simulink model "dupla_estrela_filtro_harmonico_Daniel_13mvar"  (R2023a)
settings: Solver=VariableStepAuto  StartTime=0.0  StopTime=10  FixedStep=1e-6
InitFcn:
  | r = 0.001
  | 
  | f1 = 60
  | w1 = 2 * pi * f1
  | power_bank = 13*1e6
  | voltage_bank = 34.5*1e3
  | current_bank = power_bank / (sqrt(3)*voltage_bank)
  | reactance_bank = voltage_bank^2 / power_bank
  | capacitance_bank = 1 / (w1*reactance_bank)
  | 
  | capacitance_branch = capacitance_bank / 2
  | 
  | N = 9
  | Su = 5
  | S = 2
  | 
  | C = capacitance_branch * S
  | c = C * Su / N
  | 
  | R = r * Su / N
libraries: spsSeriesRLCBranchLib x52, spsVoltageMeasurementLib x4, spsCurrentMeasurementLib x2, spsGroundLib x1, spsRMSLib x1, spsThreePhaseSourceLib x1, spspowerguiLib x1
settings Model: Creator=angel  LastModifiedBy=angel

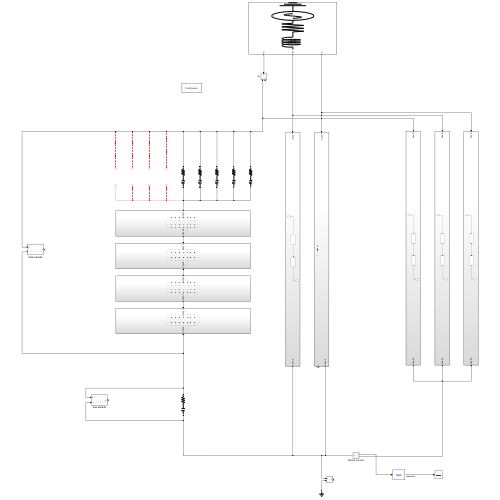
[thumbnail: Simulink's stored preview of the top-level diagram]
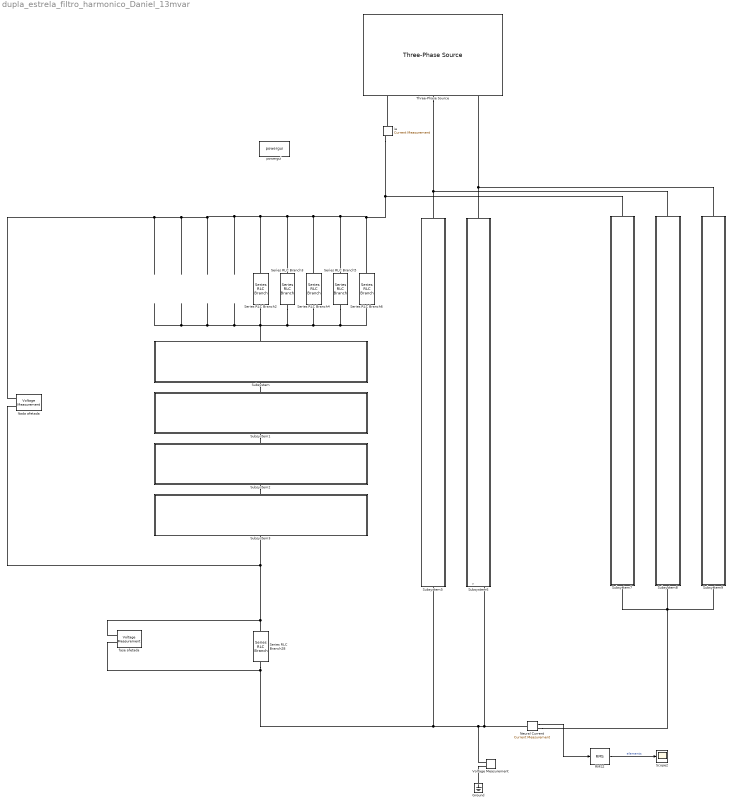
== system dupla_estrela_filtro_harmonico_Daniel_13mvar ==
  Ground : spsGroundLib/Ground  LConnTagsString=a
  Neural Current : spsCurrentMeasurementLib/Current Measurement  PhasorSimulation=off  OutputType=Complex  PSBequivalent=0
  RMS2 : spsRMSLib/RMS  TrueRMS=on  Freq=60  RMSInit=0  Ts=0
  Scope2 : Scope
  Series RLC Branch{2..6} (5 alike) : spsSeriesRLCBranchLib/Series RLC Branch  LConnTagsString=__new0  RConnTagsString=__new0  BranchType=RC  Resistance=r  Inductance=0  SetiL0=off  InitialCurrent=0  Capacitance=c  Setx0=off  InitialVoltage=0  Measurements=None
  Series RLC Branch28 : spsSeriesRLCBranchLib/Series RLC Branch  LConnTagsString=__new0  RConnTagsString=__new0  BranchType=RC  Resistance=R  Inductance=0  SetiL0=off  InitialCurrent=0  Capacitance=C  Setx0=off  InitialVoltage=0  Measurements=None
  Subsystem : Subsystem
  Subsystem1 : Subsystem
  Subsystem2 : Subsystem
  Subsystem3 : Subsystem
  Subsystem5 : Subsystem
  Subsystem6 : Subsystem
  Subsystem7 : Subsystem
  Subsystem8 : Subsystem
  Subsystem9 : Subsystem
  Three-Phase Source : spsThreePhaseSourceLib/Three-Phase Source  InternalConnection=Yg  VoltagePhases=off  Voltage=voltage_bank  PhaseAngle=0  Voltage_phases=[25e3 25e3 25e3]/sqrt(3)  PhaseAngles_phases=[0 -120 +120]  Frequency=60  NonIdealSource=on  SpecifyImpedance=off  Resistance=0.8929  Inductance=16.58e-6  ShortCircuitLevel=100e6  BaseVoltage=voltage_bank  XRratio=7  BusType=swing  Pref=10e3  Qref=0  Prefabc=[10e3, 10e3, 10e3]  Qrefabc=[0, 0, 0]  Qmin=-inf  Qmax=inf
  Voltage Measurement : spsVoltageMeasurementLib/Voltage Measurement  PhasorSimulation=off  OutputType=Complex  PSBequivalent=0
  fase afetada : spsVoltageMeasurementLib/Voltage Measurement  PhasorSimulation=off  OutputType=Complex  PSBequivalent=0
  ia : spsCurrentMeasurementLib/Current Measurement  PhasorSimulation=off  OutputType=Complex  PSBequivalent=0
  ltada afetada : spsVoltageMeasurementLib/Voltage Measurement  PhasorSimulation=off  OutputType=Complex  PSBequivalent=0
  powergui : spspowerguiLib/powergui  Priority=1  SimulationMode=Continuous  SampleTime=50e-6  frequency=60  Iterations=50  frequencyindice=60  Pbase=100e6  ErrMax=1e-4  UnitsV=kV  UnitsW=MW  buscounter=0  FunctionMessages=off  echomessages=off  EnableUseOfTLC=off  CurrentSourceSwitches=off  DisableSnubberDevices=off  DisableRonSwitches=off  DisableVfSwitches=off  DisplayEquations=off  AutomaticDiscreteSolvers=off  SolverType=Tustin/Backward Euler (TBE)  Interpol=off  ExternalGateDelay=off  methode=off  Ts=100  x0status=blocks  SPID=on  SwTol=0  HookPort=off  NonlinearTolerance=1e-4  nMaxIteration=100  ContinueOnMaxIteration=off  RestoreLinks=warning  ResistiveCurrentMeasurement=off  Frange=[0:2:500]  Ylog=off  Xlog=on  ShowGrid=off  save=off  variable=ZData  structure=0  ZoomFFT=off  StartTime=0.0  cycles=1  DisplayStyle=1  fundamental=60  FreqAxis=off  MaxFrequency=1000  frequencyindicesteady=1  RmsSteady=1  display=off
  wires:
  Neural Current/1 -> RMS2/1
  RMS2/1 -> Scope2/1  "elements"
  connections:
  Series RLC Branch6/RConn1 -- Series RLC Branch5/RConn1 -- Series RLC Branch4/RConn1 -- Series RLC Branch3/RConn1 -- Subsystem/LConn1 -- Series RLC Branch2/RConn1
  ltada afetada/LConn1 -- Series RLC Branch2/LConn1 -- Series RLC Branch3/LConn1 -- Series RLC Branch4/LConn1 -- Series RLC Branch5/LConn1 -- Subsystem7/LConn1 -- ia/RConn1 -- Series RLC Branch6/LConn1
  Three-Phase Source/RConn2 -- Subsystem8/LConn1 -- Subsystem5/LConn1
  fase afetada/LConn2 -- Series RLC Branch28/RConn1 -- Subsystem5/RConn1 -- Subsystem6/RConn1 -- Neural Current/LConn1 -- Voltage Measurement/LConn1
  Subsystem/RConn1 -- Subsystem1/LConn1
  Subsystem1/RConn1 -- Subsystem2/LConn1
  Subsystem2/RConn1 -- Subsystem3/LConn1
  Series RLC Branch28/LConn1 -- ltada afetada/LConn2 -- Subsystem3/RConn1 -- fase afetada/LConn1
  Three-Phase Source/RConn3 -- Subsystem6/LConn1 -- Subsystem9/LConn1
  Neural Current/RConn1 -- Subsystem9/RConn1 -- Subsystem8/RConn1 -- Subsystem7/RConn1
  ia/LConn1 -- Three-Phase Source/RConn1
  Ground/LConn1 -- Voltage Measurement/LConn2

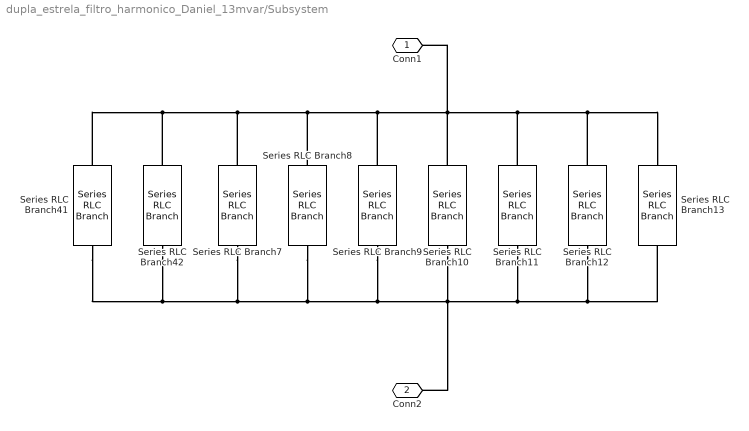
== system dupla_estrela_filtro_harmonico_Daniel_13mvar/Subsystem ==
  Series RLC Branch{7..13,41..42} (9 alike) : spsSeriesRLCBranchLib/Series RLC Branch  LConnTagsString=__new0  RConnTagsString=__new0  BranchType=RC  Resistance=r  Inductance=0  SetiL0=off  InitialCurrent=0  Capacitance=c  Setx0=off  InitialVoltage=0  Measurements=None
  Conn1 : PMIOPort  Side=Left
  Conn2 : PMIOPort  Port=2  Side=Right
  connections:
  Series RLC Branch42/LConn1 -- Series RLC Branch8/LConn1 -- Series RLC Branch9/LConn1 -- Conn1/RConn1 -- Series RLC Branch11/LConn1 -- Series RLC Branch12/LConn1 -- Series RLC Branch13/LConn1 -- Series RLC Branch10/LConn1 -- Series RLC Branch7/LConn1 -- Series RLC Branch41/LConn1
  Series RLC Branch42/RConn1 -- Series RLC Branch7/RConn1 -- Conn2/RConn1 -- Series RLC Branch13/RConn1 -- Series RLC Branch12/RConn1 -- Series RLC Branch11/RConn1 -- Series RLC Branch10/RConn1 -- Series RLC Branch9/RConn1 -- Series RLC Branch8/RConn1 -- Series RLC Branch41/RConn1

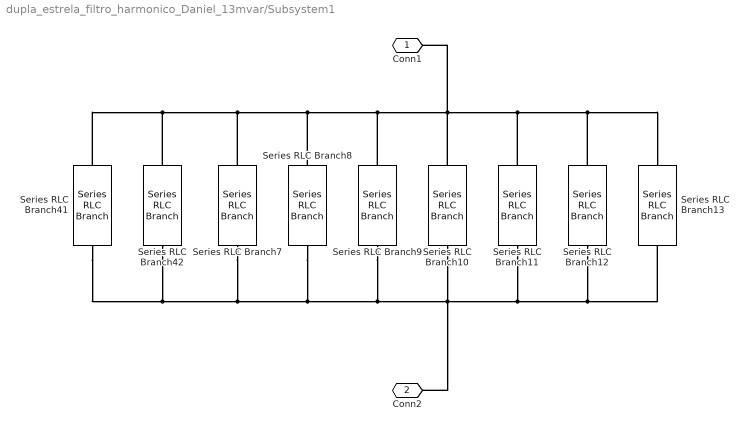
== system dupla_estrela_filtro_harmonico_Daniel_13mvar/Subsystem1 ==
  Series RLC Branch{7..13,41..42} (9 alike) : spsSeriesRLCBranchLib/Series RLC Branch  LConnTagsString=__new0  RConnTagsString=__new0  BranchType=RC  Resistance=r  Inductance=0  SetiL0=off  InitialCurrent=0  Capacitance=c  Setx0=off  InitialVoltage=0  Measurements=None
  Conn1 : PMIOPort  Side=Left
  Conn2 : PMIOPort  Port=2  Side=Right
  connections:
  Conn2/RConn1 -- Series RLC Branch10/RConn1 -- Series RLC Branch9/RConn1 -- Series RLC Branch8/RConn1 -- Series RLC Branch42/RConn1 -- Series RLC Branch41/RConn1 -- Series RLC Branch7/RConn1 -- Series RLC Branch11/RConn1 -- Series RLC Branch12/RConn1 -- Series RLC Branch13/RConn1
  Conn1/RConn1 -- Series RLC Branch10/LConn1 -- Series RLC Branch13/LConn1 -- Series RLC Branch12/LConn1 -- Series RLC Branch11/LConn1 -- Series RLC Branch9/LConn1 -- Series RLC Branch8/LConn1 -- Series RLC Branch7/LConn1 -- Series RLC Branch41/LConn1 -- Series RLC Branch42/LConn1

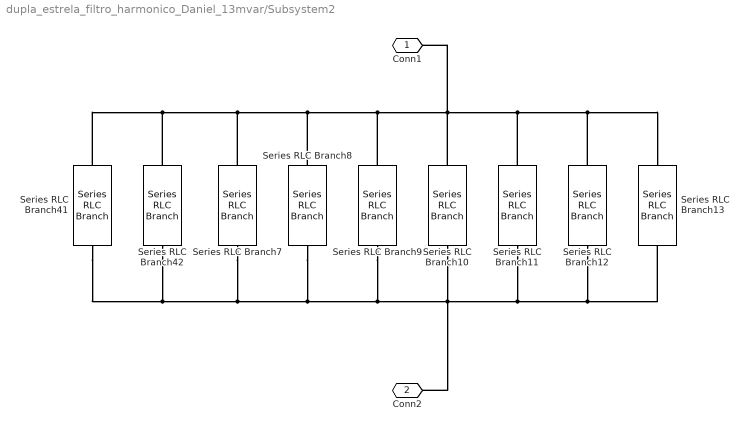
== system dupla_estrela_filtro_harmonico_Daniel_13mvar/Subsystem2 ==
  Series RLC Branch{7..13,41..42} (9 alike) : spsSeriesRLCBranchLib/Series RLC Branch  LConnTagsString=__new0  RConnTagsString=__new0  BranchType=RC  Resistance=r  Inductance=0  SetiL0=off  InitialCurrent=0  Capacitance=c  Setx0=off  InitialVoltage=0  Measurements=None
  Conn1 : PMIOPort  Side=Left
  Conn2 : PMIOPort  Port=2  Side=Right
  connections:
  Series RLC Branch42/LConn1 -- Series RLC Branch41/LConn1 -- Series RLC Branch7/LConn1 -- Series RLC Branch8/LConn1 -- Series RLC Branch9/LConn1 -- Series RLC Branch11/LConn1 -- Series RLC Branch12/LConn1 -- Series RLC Branch13/LConn1 -- Series RLC Branch10/LConn1 -- Conn1/RConn1
  Series RLC Branch13/RConn1 -- Series RLC Branch12/RConn1 -- Series RLC Branch11/RConn1 -- Series RLC Branch7/RConn1 -- Series RLC Branch41/RConn1 -- Series RLC Branch42/RConn1 -- Series RLC Branch8/RConn1 -- Series RLC Branch9/RConn1 -- Series RLC Branch10/RConn1 -- Conn2/RConn1

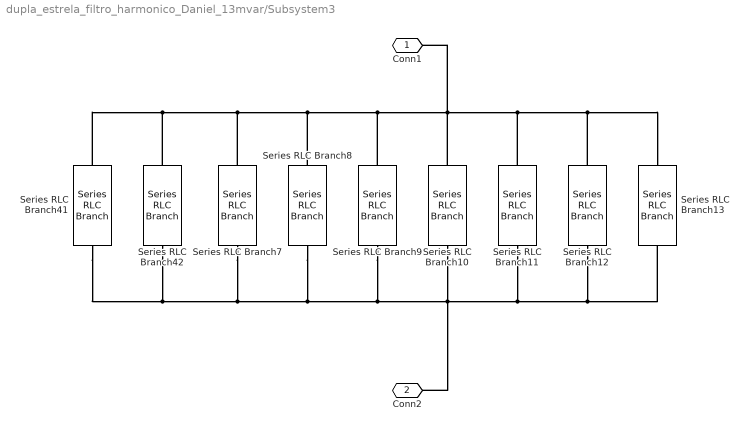
== system dupla_estrela_filtro_harmonico_Daniel_13mvar/Subsystem3 ==
  Series RLC Branch{7..13,41..42} (9 alike) : spsSeriesRLCBranchLib/Series RLC Branch  LConnTagsString=__new0  RConnTagsString=__new0  BranchType=RC  Resistance=r  Inductance=0  SetiL0=off  InitialCurrent=0  Capacitance=c  Setx0=off  InitialVoltage=0  Measurements=None
  Conn1 : PMIOPort  Side=Left
  Conn2 : PMIOPort  Port=2  Side=Right
  connections:
  Conn2/RConn1 -- Series RLC Branch10/RConn1 -- Series RLC Branch9/RConn1 -- Series RLC Branch8/RConn1 -- Series RLC Branch42/RConn1 -- Series RLC Branch41/RConn1 -- Series RLC Branch7/RConn1 -- Series RLC Branch11/RConn1 -- Series RLC Branch12/RConn1 -- Series RLC Branch13/RConn1
  Conn1/RConn1 -- Series RLC Branch10/LConn1 -- Series RLC Branch13/LConn1 -- Series RLC Branch12/LConn1 -- Series RLC Branch11/LConn1 -- Series RLC Branch9/LConn1 -- Series RLC Branch8/LConn1 -- Series RLC Branch7/LConn1 -- Series RLC Branch41/LConn1 -- Series RLC Branch42/LConn1

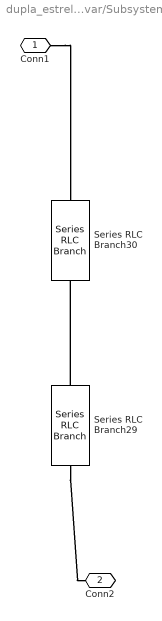
== system dupla_estrela_filtro_harmonico_Daniel_13mvar/Subsystem5 ==
  Series RLC Branch29 : spsSeriesRLCBranchLib/Series RLC Branch  LConnTagsString=__new0  RConnTagsString=__new0  BranchType=RC  Resistance=R  Inductance=0  SetiL0=off  InitialCurrent=0  Capacitance=C  Setx0=off  InitialVoltage=0  Measurements=None
  Series RLC Branch30 : spsSeriesRLCBranchLib/Series RLC Branch  LConnTagsString=__new0  RConnTagsString=__new0  BranchType=RC  Resistance=R  Inductance=0  SetiL0=off  InitialCurrent=0  Capacitance=C  Setx0=off  InitialVoltage=0  Measurements=None
  Conn1 : PMIOPort  Side=Left
  Conn2 : PMIOPort  Port=2  Side=Right
  connections:
  Series RLC Branch29/LConn1 -- Series RLC Branch30/RConn1
  Series RLC Branch29/RConn1 -- Conn2/RConn1
  Conn1/RConn1 -- Series RLC Branch30/LConn1

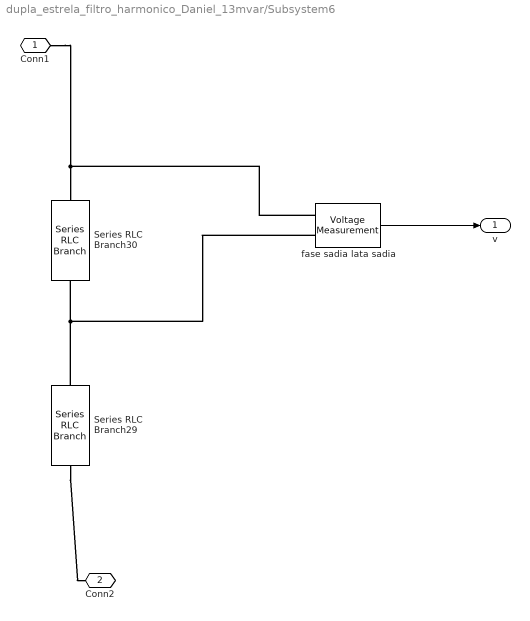
== system dupla_estrela_filtro_harmonico_Daniel_13mvar/Subsystem6 ==
  Series RLC Branch29 : spsSeriesRLCBranchLib/Series RLC Branch  LConnTagsString=__new0  RConnTagsString=__new0  BranchType=RC  Resistance=R  Inductance=0  SetiL0=off  InitialCurrent=0  Capacitance=C  Setx0=off  InitialVoltage=0  Measurements=None
  Series RLC Branch30 : spsSeriesRLCBranchLib/Series RLC Branch  LConnTagsString=__new0  RConnTagsString=__new0  BranchType=RC  Resistance=R  Inductance=0  SetiL0=off  InitialCurrent=0  Capacitance=C  Setx0=off  InitialVoltage=0  Measurements=None
  fase sadia lata sadia : spsVoltageMeasurementLib/Voltage Measurement  PhasorSimulation=off  OutputType=Complex  PSBequivalent=0
  Conn1 : PMIOPort  Side=Left
  Conn2 : PMIOPort  Port=2  Side=Right
  v : Outport
  wires:
  fase sadia lata sadia/1 -> v/1
  connections:
  Conn1/RConn1 -- fase sadia lata sadia/LConn1 -- Series RLC Branch30/LConn1
  Series RLC Branch29/RConn1 -- Conn2/RConn1
  Series RLC Branch29/LConn1 -- fase sadia lata sadia/LConn2 -- Series RLC Branch30/RConn1

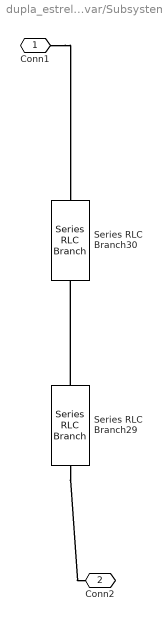
== system dupla_estrela_filtro_harmonico_Daniel_13mvar/Subsystem7 ==
  Series RLC Branch29 : spsSeriesRLCBranchLib/Series RLC Branch  LConnTagsString=__new0  RConnTagsString=__new0  BranchType=RC  Resistance=R  Inductance=0  SetiL0=off  InitialCurrent=0  Capacitance=C  Setx0=off  InitialVoltage=0  Measurements=None
  Series RLC Branch30 : spsSeriesRLCBranchLib/Series RLC Branch  LConnTagsString=__new0  RConnTagsString=__new0  BranchType=RC  Resistance=R  Inductance=0  SetiL0=off  InitialCurrent=0  Capacitance=C  Setx0=off  InitialVoltage=0  Measurements=None
  Conn1 : PMIOPort  Side=Left
  Conn2 : PMIOPort  Port=2  Side=Right
  connections:
  Series RLC Branch29/LConn1 -- Series RLC Branch30/RConn1
  Series RLC Branch29/RConn1 -- Conn2/RConn1
  Conn1/RConn1 -- Series RLC Branch30/LConn1

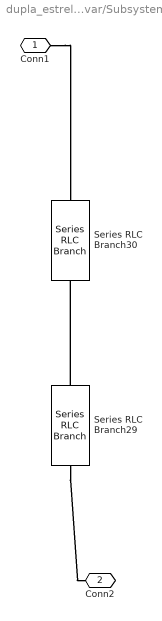
== system dupla_estrela_filtro_harmonico_Daniel_13mvar/Subsystem8 ==
  Series RLC Branch29 : spsSeriesRLCBranchLib/Series RLC Branch  LConnTagsString=__new0  RConnTagsString=__new0  BranchType=RC  Resistance=R  Inductance=0  SetiL0=off  InitialCurrent=0  Capacitance=C  Setx0=off  InitialVoltage=0  Measurements=None
  Series RLC Branch30 : spsSeriesRLCBranchLib/Series RLC Branch  LConnTagsString=__new0  RConnTagsString=__new0  BranchType=RC  Resistance=R  Inductance=0  SetiL0=off  InitialCurrent=0  Capacitance=C  Setx0=off  InitialVoltage=0  Measurements=None
  Conn1 : PMIOPort  Side=Left
  Conn2 : PMIOPort  Port=2  Side=Right
  connections:
  Conn1/RConn1 -- Series RLC Branch30/LConn1
  Series RLC Branch29/RConn1 -- Conn2/RConn1
  Series RLC Branch29/LConn1 -- Series RLC Branch30/RConn1

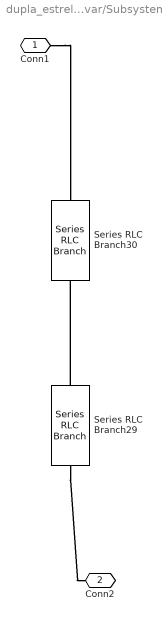
== system dupla_estrela_filtro_harmonico_Daniel_13mvar/Subsystem9 ==
  Series RLC Branch29 : spsSeriesRLCBranchLib/Series RLC Branch  LConnTagsString=__new0  RConnTagsString=__new0  BranchType=RC  Resistance=R  Inductance=0  SetiL0=off  InitialCurrent=0  Capacitance=C  Setx0=off  InitialVoltage=0  Measurements=None
  Series RLC Branch30 : spsSeriesRLCBranchLib/Series RLC Branch  LConnTagsString=__new0  RConnTagsString=__new0  BranchType=RC  Resistance=R  Inductance=0  SetiL0=off  InitialCurrent=0  Capacitance=C  Setx0=off  InitialVoltage=0  Measurements=None
  Conn1 : PMIOPort  Side=Left
  Conn2 : PMIOPort  Port=2  Side=Right
  connections:
  Series RLC Branch29/LConn1 -- Series RLC Branch30/RConn1
  Series RLC Branch29/RConn1 -- Conn2/RConn1
  Conn1/RConn1 -- Series RLC Branch30/LConn1
